simulink model "icecast_modelo"  (R2015a)
settings: Solver=FixedStepDiscrete  StartTime=0.0  StopTime=1000  FixedStep=0.1  RelTol=1e-3
settings Model: Creator=windor  LastModifiedBy=windor

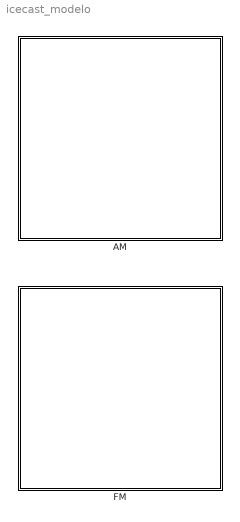
== system icecast_modelo ==
  AM : Subsystem
  FM : Subsystem

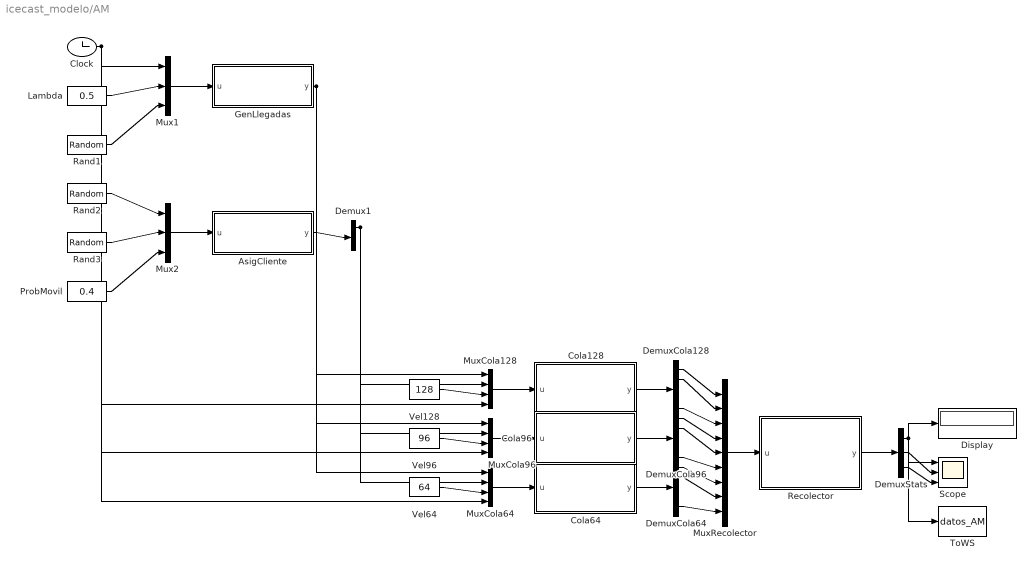
== system icecast_modelo/AM ==
  AsigCliente : MATLAB Function  TreatAsAtomicUnit=on
  Clock : Clock
  Cola128 : MATLAB Function  TreatAsAtomicUnit=on
  Cola64 : MATLAB Function  TreatAsAtomicUnit=on
  Cola96 : MATLAB Function  TreatAsAtomicUnit=on
  Demux1 : Demux  Outputs=2
  DemuxCola128 : Demux  Outputs=5
  DemuxCola64 : Demux  Outputs=5
  DemuxCola96 : Demux  Outputs=5
  DemuxStats : Demux  Outputs=3
  Display : Display
  GenLlegadas : MATLAB Function  TreatAsAtomicUnit=on
  Lambda : Constant  Value=0.5
  Mux1 : Mux  Inputs=3
  Mux2 : Mux  Inputs=3
  MuxCola128 : Mux
  MuxCola64 : Mux
  MuxCola96 : Mux
  MuxRecolector : Mux  Inputs=9
  ProbMovil : Constant  Value=0.4
  Rand1 : UniformRandomNumber  Seed=1  SampleTime=0.1
  Rand2 : UniformRandomNumber  Seed=2  SampleTime=0.1
  Rand3 : UniformRandomNumber  Seed=3  SampleTime=0.1
  Recolector : MATLAB Function  TreatAsAtomicUnit=on
  Scope : Scope  NumInputPorts=3
  ToWS : ToWorkspace  VariableName=datos_AM  SaveFormat=Structure  SampleTime=-1
  Vel128 : Constant  Value=128
  Vel64 : Constant  Value=64
  Vel96 : Constant  Value=96
  wires:
  Clock/1 -> Mux1/1, MuxCola128/4, MuxCola96/4, MuxCola64/4
  Lambda/1 -> Mux1/2
  Rand1/1 -> Mux1/3
  Mux1/1 -> GenLlegadas/1(u)
  Rand2/1 -> Mux2/1
  Rand3/1 -> Mux2/2
  ProbMovil/1 -> Mux2/3
  Mux2/1 -> AsigCliente/1(u)
  AsigCliente/1(y) -> Demux1/1
  GenLlegadas/1(y) -> MuxCola128/1, MuxCola96/1, MuxCola64/1
  Demux1/1 -> MuxCola128/2, MuxCola96/2, MuxCola64/2
  Vel128/1 -> MuxCola128/3
  MuxCola128/1 -> Cola128/1(u)
  Cola128/1(y) -> DemuxCola128/1
  Vel96/1 -> MuxCola96/3
  MuxCola96/1 -> Cola96/1(u)
  Cola96/1(y) -> DemuxCola96/1
  Vel64/1 -> MuxCola64/3
  MuxCola64/1 -> Cola64/1(u)
  Cola64/1(y) -> DemuxCola64/1
  DemuxCola128/1 -> MuxRecolector/1
  DemuxCola128/2 -> MuxRecolector/2
  DemuxCola128/5 -> MuxRecolector/3
  DemuxCola96/1 -> MuxRecolector/4
  DemuxCola96/2 -> MuxRecolector/5
  DemuxCola96/5 -> MuxRecolector/6
  DemuxCola64/1 -> MuxRecolector/7
  DemuxCola64/2 -> MuxRecolector/8
  DemuxCola64/5 -> MuxRecolector/9
  MuxRecolector/1 -> Recolector/1(u)
  Recolector/1(y) -> DemuxStats/1
  DemuxStats/1 -> Display/1, Scope/1, ToWS/1
  DemuxStats/2 -> Scope/2
  DemuxStats/3 -> Scope/3

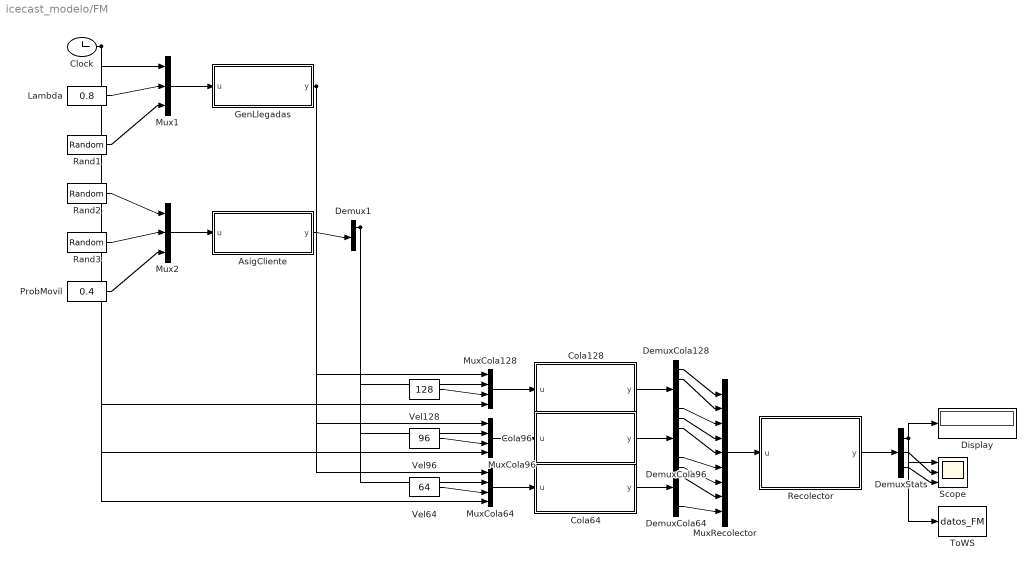
== system icecast_modelo/FM ==
  AsigCliente : MATLAB Function  TreatAsAtomicUnit=on
  Clock : Clock
  Cola128 : MATLAB Function  TreatAsAtomicUnit=on
  Cola64 : MATLAB Function  TreatAsAtomicUnit=on
  Cola96 : MATLAB Function  TreatAsAtomicUnit=on
  Demux1 : Demux  Outputs=2
  DemuxCola128 : Demux  Outputs=5
  DemuxCola64 : Demux  Outputs=5
  DemuxCola96 : Demux  Outputs=5
  DemuxStats : Demux  Outputs=3
  Display : Display
  GenLlegadas : MATLAB Function  TreatAsAtomicUnit=on
  Lambda : Constant  Value=0.8
  Mux1 : Mux  Inputs=3
  Mux2 : Mux  Inputs=3
  MuxCola128 : Mux
  MuxCola64 : Mux
  MuxCola96 : Mux
  MuxRecolector : Mux  Inputs=9
  ProbMovil : Constant  Value=0.4
  Rand1 : UniformRandomNumber  Seed=1  SampleTime=0.1
  Rand2 : UniformRandomNumber  Seed=2  SampleTime=0.1
  Rand3 : UniformRandomNumber  Seed=3  SampleTime=0.1
  Recolector : MATLAB Function  TreatAsAtomicUnit=on
  Scope : Scope  NumInputPorts=3
  ToWS : ToWorkspace  VariableName=datos_FM  SaveFormat=Structure  SampleTime=-1
  Vel128 : Constant  Value=128
  Vel64 : Constant  Value=64
  Vel96 : Constant  Value=96
  wires:
  DemuxStats/3 -> Scope/3
  DemuxStats/2 -> Scope/2
  DemuxStats/1 -> ToWS/1, Scope/1, Display/1
  Recolector/1(y) -> DemuxStats/1
  MuxRecolector/1 -> Recolector/1(u)
  DemuxCola64/5 -> MuxRecolector/9
  DemuxCola64/2 -> MuxRecolector/8
  DemuxCola64/1 -> MuxRecolector/7
  DemuxCola96/5 -> MuxRecolector/6
  DemuxCola96/2 -> MuxRecolector/5
  DemuxCola96/1 -> MuxRecolector/4
  DemuxCola128/5 -> MuxRecolector/3
  DemuxCola128/2 -> MuxRecolector/2
  DemuxCola128/1 -> MuxRecolector/1
  Cola64/1(y) -> DemuxCola64/1
  MuxCola64/1 -> Cola64/1(u)
  Vel64/1 -> MuxCola64/3
  Cola96/1(y) -> DemuxCola96/1
  MuxCola96/1 -> Cola96/1(u)
  Vel96/1 -> MuxCola96/3
  Cola128/1(y) -> DemuxCola128/1
  MuxCola128/1 -> Cola128/1(u)
  Vel128/1 -> MuxCola128/3
  Demux1/1 -> MuxCola64/2, MuxCola96/2, MuxCola128/2
  GenLlegadas/1(y) -> MuxCola64/1, MuxCola96/1, MuxCola128/1
  AsigCliente/1(y) -> Demux1/1
  Mux2/1 -> AsigCliente/1(u)
  ProbMovil/1 -> Mux2/3
  Rand3/1 -> Mux2/2
  Rand2/1 -> Mux2/1
  Mux1/1 -> GenLlegadas/1(u)
  Rand1/1 -> Mux1/3
  Lambda/1 -> Mux1/2
  Clock/1 -> MuxCola64/4, MuxCola96/4, MuxCola128/4, Mux1/1

== matlab function icecast_modelo/AM/AsigCliente ==
  data: u input; y output
function y = fcn(u)
%#codegen

y = u;

== matlab function icecast_modelo/AM/GenLlegadas ==
  data: u input; y output
function y = fcn(u)
%#codegen

y = u;

== matlab function icecast_modelo/AM/Cola128 ==
  data: u input; y output
function y = fcn(u)
%#codegen

y = u;

== matlab function icecast_modelo/AM/Cola96 ==
  data: u input; y output
function y = fcn(u)
%#codegen

y = u;

== matlab function icecast_modelo/AM/Cola64 ==
  data: u input; y output
function y = fcn(u)
%#codegen

y = u;

== matlab function icecast_modelo/AM/Recolector ==
  data: u input; y output
function y = fcn(u)
%#codegen

y = u;

== matlab function icecast_modelo/FM/AsigCliente ==
  data: u input; y output
function y = fcn(u)
%#codegen

y = u;

== matlab function icecast_modelo/FM/Cola128 ==
  data: u input; y output
function y = fcn(u)
%#codegen

y = u;

== matlab function icecast_modelo/FM/Cola64 ==
  data: u input; y output
function y = fcn(u)
%#codegen

y = u;

== matlab function icecast_modelo/FM/Cola96 ==
  data: u input; y output
function y = fcn(u)
%#codegen

y = u;

== matlab function icecast_modelo/FM/GenLlegadas ==
  data: u input; y output
function y = fcn(u)
%#codegen

y = u;

== matlab function icecast_modelo/FM/Recolector ==
  data: u input; y output
function y = fcn(u)
%#codegen

y = u;
